simulink model "NeuromuscularModel"  (R2019b)
settings: Solver=ode15s  StartTime=0.0  StopTime=inf  MaxStep=.01  RelTol=1e-4  AbsTol=1e-6  EnableMultiTasking=on
values from neighbouring files (symbols this model uses):
  LceOffsetTA = 1-0.5*w    [ControlParams.m]
  legAngleTgt = 1.2    [ControlParams.m]    (also in assignGains.m = Gains(45))
  LongDelay = 0.020    (= 0.02)    [ControlParams.m]
  MidDelay = 0.010    (= 0.01)    [ControlParams.m]
  ShortDelay = 0.005    [ControlParams.m]
  simbiconGainD = 5*pi/180    (= 0.0872664625997)    [ControlParams.m]    (also in assignGains.m = Gains(42))
  simbiconGainV = 5*pi/180    (= 0.0872664625997)    [ControlParams.m]    (also in assignGains.m = Gains(43))
  simbiconLegAngle0 = 85*pi/180    (= 1.4835298642)    [ControlParams.m]    (also in assignGains.m = Gains(44))
undefined symbols (not defined in the file or in its folder): footCenterToCGDist, footInertia, footMass, g, legLengthClr, loptGAS, loptTA, lslackGAS, phimaxGASa, phimaxGASk, phirefGASa, phirefGASk, rGASa, rGASk, rhoGASa, rhoGASk, X, Y, Z
libraries: NeuroMuscularLibrary x81, nesl_utility x22, sm_lib x16, simulink x4, simulink_extras x2
(part 2 of 2)

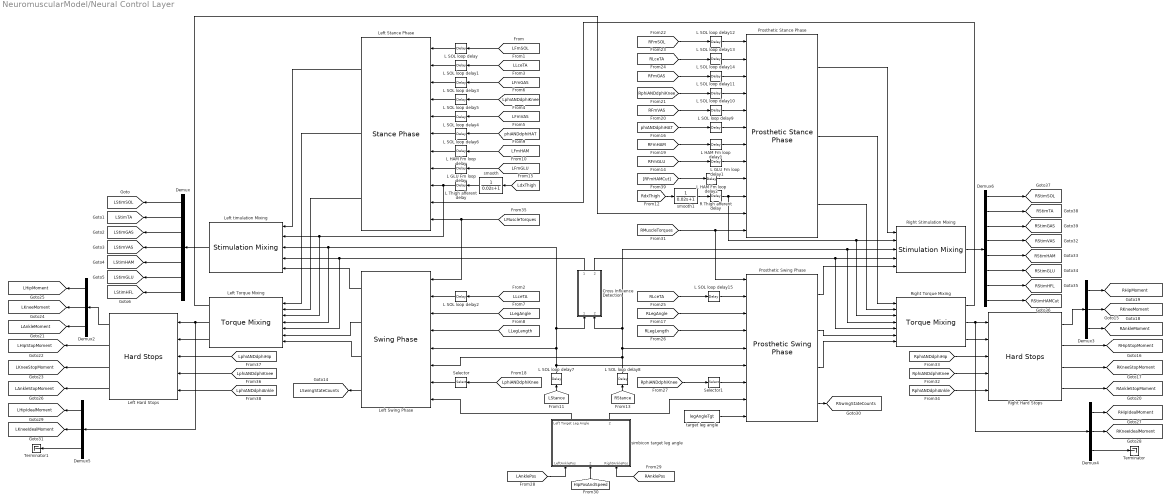
== system NeuromuscularModel/Neural Control Layer ==
  Cross Influence Detection : Subsystem
  Demux : Demux  Outputs=7
  Demux{2..5} (4 alike) : Demux  Outputs=3
  Demux6 : Demux  Outputs=8
  L GLU Fm loop delay : TransportDelay  DelayTime=ShortDelay
  L GLU Fm loop delay1 : TransportDelay  DelayTime=ShortDelay
  L HAM Fm loop delay : TransportDelay  DelayTime=ShortDelay
  L HAM Fm loop delay1 : TransportDelay  DelayTime=ShortDelay
  L HAM Fm loop delay2 : TransportDelay  DelayTime=ShortDelay  BufferSize=2048
  L SOL loop delay{,1..3,12..15} (8 alike) : TransportDelay  DelayTime=LongDelay
  L SOL loop delay{4..5,7..8,10..11} (6 alike) : TransportDelay  DelayTime=MidDelay
  L SOL loop delay6 : TransportDelay  DelayTime=ShortDelay
  L SOL loop delay9 : TransportDelay  DelayTime=ShortDelay
  L Thigh afferent delay : TransportDelay  DelayTime=ShortDelay
  Left Hard Stops : NeuroMuscularLibrary/Hard Stops  SystemSampleTime=-1  Latency=0  AutoFrameSizeCalculation=off
  Left Stance Phase : NeuroMuscularLibrary/Stance Phase  GainHAM=LGainHAM  GainGLU=LGainGLU  GainSOL=LGainSOL  GainSOLTA=LGainSOLTA  GainTA=LGainTA  GainGAS=LGainGAS  GainVAS=LGainVAS  GainKneeOverExt=LGainKneeOverExt  PosGainGG=LPosGainGG  SpeedGainGG=LSpeedGainGG  Kglu=LKglu
  Left Swing Phase : NeuroMuscularLibrary/Swing Phase  GainTA=LGainTA  hipPGain=LhipPGain  hipDGain=LhipDGain  legAngleFilter=LlegAngleFilter  kneeFlexGain=LkneeFlexGain  kneeHoldGain1=LkneeHoldGain1  kneeHoldGain2=LkneeHoldGain2  kneeStopGain=LkneeStopGain  kneeExtendGain=LkneeExtendGain  legLengthClr=LlegLengthClr
  Left Torque Mixing : NeuroMuscularLibrary/Torque Mixing  SystemSampleTime=-1  Latency=0  AutoFrameSizeCalculation=off
  Left timulation Mixing : NeuroMuscularLibrary/Stimulation Mixing  SystemSampleTime=-1  Latency=0  AutoFrameSizeCalculation=off
  Prosthetic Stance Phase : NeuroMuscularLibrary/Prosthetic Stance Phase  GainHAM=RGainHAM  GainHAMCut=RGainHAMCut  GainGLU=RGainGLU  GainSOL=RGainSOL  GainSOLTA=RGainSOLTA  GainTA=RGainTA  GainGAS=RGainGAS  GainVAS=RGainVAS  GainKneeOverExt=RGainKneeOverExt  PosGainGG=RPosGainGG  SpeedGainGG=RSpeedGainGG  Kglu=RKglu
  Prosthetic Swing Phase : NeuroMuscularLibrary/Prosthetic Swing Phase  GainTA=RGainTA  hipPGain=RhipPGain  hipDGain=RhipDGain  legAngleFilter=RlegAngleFilter  kneeFlexGain=RkneeFlexGain  kneeHoldGain1=RkneeHoldGain1  kneeHoldGain2=RkneeHoldGain2  kneeStopGain=RkneeStopGain  kneeExtendGain=RkneeExtendGain  legLengthClr=RlegLengthClr
  R Thigh afferent delay : TransportDelay  DelayTime=ShortDelay
  Right Hard Stops : NeuroMuscularLibrary/Hard Stops  SystemSampleTime=-1  Latency=0  AutoFrameSizeCalculation=off
  Right Stimulation Mixing : NeuroMuscularLibrary/Stimulation Mixing  SystemSampleTime=-1  Latency=0  AutoFrameSizeCalculation=off
  Right Torque Mixing : NeuroMuscularLibrary/Torque Mixing  SystemSampleTime=-1  Latency=0  AutoFrameSizeCalculation=off
  Selector : Selector  InputPortWidth=2  IndexOptions=Index vector (dialog)  Indices=2  OutputSizes=1
  Selector1 : Selector  InputPortWidth=2  IndexOptions=Index vector (dialog)  Indices=2  OutputSizes=1
  Terminator : Terminator
  Terminator1 : Terminator
  simbicon target leg angle : Subsystem
  smooth : TransferFcn  Denominator=[0.02 1]
  smooth1 : TransferFcn  Denominator=[0.02 1]
  target leg angle : Constant  Value=legAngleTgt
  tag scope: LAnkleMoment=global, LAnkleStopMoment=global, LHipIdealMoment=global, LHipMoment=global, LHipStopMoment=global, LKneeIdealMoment=global, LKneeMoment=global, LKneeStopMoment=global, LStimGAS=global, LStimGLU=global, LStimHAM=global, LStimHFL=global, LStimSOL=global, LStimTA=global, LStimVAS=global, LSwingStateCounts=global, RAnkleMoment=global, RAnkleStopMoment=global, RHipIdealMoment=global, RHipMoment=global, RHipStopMoment=global, RKneeIdealMoment=global, RKneeMoment=global, RKneeStopMoment=global, RStimGAS=global, RStimGLU=global, RStimHAM=global, RStimHAMCut=global, RStimHFL=global, RStimSOL=global, RStimTA=global, RStimVAS=global, RSwingStateCounts=global
  wires:
  target leg angle/1 -> Prosthetic Swing Phase/9
  L HAM Fm loop delay2/1 -> Prosthetic Stance Phase/9
  [RFmHAMCut] -> L HAM Fm loop delay2/1
  L GLU Fm loop delay1/1 -> Prosthetic Stance Phase/8
  L HAM Fm loop delay1/1 -> Prosthetic Stance Phase/7
  Demux6/8 -> [RStimHAMCut]
  Right Stimulation Mixing/1 -> Demux6/1
  Demux6/6 -> [RStimGLU]
  Demux6/3 -> [RStimGAS]
  Demux6/7 -> [RStimHFL]
  Demux6/5 -> [RStimHAM]
  Demux6/4 -> [RStimVAS]
  Demux6/2 -> [RStimTA]
  Demux6/1 -> [RStimSOL]
  Demux5/3 -> Terminator1/1
  Demux5/2 -> [LKneeIdealMoment]
  Demux5/1 -> [LHipIdealMoment]
  Left Swing Phase/3 -> Left Torque Mixing/7
  Left Swing Phase/2 -> Left Torque Mixing/6
  Left Stance Phase/3 -> Left Torque Mixing/2
  Left Torque Mixing/1 -> Prosthetic Stance Phase/11
  Left Torque Mixing/3 -> Left Hard Stops/2
  Left Torque Mixing/2 -> Left Hard Stops/1, Demux5/1
  [LphiANDdphiAnkle] -> Left Hard Stops/5
  Right Torque Mixing/1 -> Left Stance Phase/10
  Right Torque Mixing/3 -> Right Hard Stops/2
  Prosthetic Stance Phase/2 -> Right Torque Mixing/1
  Prosthetic Stance Phase/3 -> Right Torque Mixing/2
  Prosthetic Swing Phase/2 -> Right Torque Mixing/6
  Prosthetic Swing Phase/3 -> Right Torque Mixing/7
  Demux4/3 -> Terminator/1
  Demux4/2 -> [RKneeIdealMoment]
  Demux4/1 -> [RHipIdealMoment]
  [RMuscleTorques] -> Prosthetic Swing Phase/1, Prosthetic Stance Phase/12
  Right Hard Stops/1 -> Demux3/1
  Right Torque Mixing/2 -> Right Hard Stops/1, Demux4/1
  Demux2/2 -> [LKneeMoment]
  Left Stance Phase/2 -> Left Torque Mixing/1
  Left Hard Stops/4 -> [LAnkleStopMoment]
  Left Hard Stops/3 -> [LKneeStopMoment]
  Left Hard Stops/2 -> [LHipStopMoment]
  [LphiANDdphiHip] -> Left Hard Stops/3
  [LphiANDdphiKnee] -> Left Hard Stops/4
  Left Hard Stops/1 -> Demux2/1
  Demux2/3 -> [LAnkleMoment]
  Demux2/1 -> [LHipMoment]
  [LMuscleTorques] -> Left Stance Phase/11, Left Swing Phase/1
  Right Hard Stops/4 -> [RAnkleStopMoment]
  Right Hard Stops/3 -> [RKneeStopMoment]
  Right Hard Stops/2 -> [RHipStopMoment]
  [RphiANDdphiAnkle] -> Right Hard Stops/5
  [RphiANDdphiHip] -> Right Hard Stops/3
  [RphiANDdphiKnee] -> Right Hard Stops/4
  Demux3/3 -> [RAnkleMoment]
  Left Swing Phase/4 -> [LSwingStateCounts]
  Prosthetic Swing Phase/4 -> [RSwingStateCounts]
  simbicon target leg angle/1(Left Target Leg Angle) -> Left Swing Phase/8
  simbicon target leg angle/2(Right Target Leg Angle) -> Prosthetic Swing Phase/8
  [HipPosAndSpeed] -> simbicon target leg angle/2(HIPposAndSpeed)
  Left Swing Phase/1 -> Left timulation Mixing/5
  Selector/1 -> Left Swing Phase/7
  [LphiANDdphiKnee] -> Selector/1
  Prosthetic Swing Phase/1 -> Right Stimulation Mixing/5
  [RAnklePos] -> simbicon target leg angle/3(RightAnklePos)
  [LAnklePos] -> simbicon target leg angle/1(LeftAnklePos)
  Selector1/1 -> Prosthetic Swing Phase/7
  [RphiANDdphiKnee] -> Selector1/1
  [RLegLength] -> Prosthetic Swing Phase/4
  [RLegAngle] -> Prosthetic Swing Phase/3
  [LLegLength] -> Left Swing Phase/4
  [LLegAngle] -> Left Swing Phase/3
  Demux3/2 -> [RKneeMoment]
  Demux3/1 -> [RHipMoment]
  Cross Influence Detection/1(RightLeading) -> Left timulation Mixing/4, Left Torque Mixing/5
  Left Stance Phase/1 -> Left timulation Mixing/1
  Left timulation Mixing/1 -> Demux/1
  Cross Influence Detection/2(LeftLeading) -> Right Stimulation Mixing/4, Right Torque Mixing/5
  L SOL loop delay8/1 -> Cross Influence Detection/2(RStance), Right Stimulation Mixing/3, Right Torque Mixing/4, Prosthetic Swing Phase/5, Left Swing Phase/6
  Prosthetic Stance Phase/1 -> Right Stimulation Mixing/1
  L SOL loop delay2/1 -> Left Swing Phase/2
  L SOL loop delay15/1 -> Prosthetic Swing Phase/2
  R Thigh afferent delay/1 -> Right Stimulation Mixing/2, Right Torque Mixing/3, Prosthetic Stance Phase/10
  L GLU Fm loop delay/1 -> Left Stance Phase/8
  L HAM Fm loop delay/1 -> Left Stance Phase/7
  L Thigh afferent delay/1 -> Left Stance Phase/9, Left timulation Mixing/2, Left Torque Mixing/3
  [RLceTA] -> L SOL loop delay15/1
  L SOL loop delay14/1 -> Prosthetic Stance Phase/3
  [RFmGAS] -> L SOL loop delay14/1
  L SOL loop delay13/1 -> Prosthetic Stance Phase/2
  [RLceTA] -> L SOL loop delay13/1
  [RFmSOL] -> L SOL loop delay12/1
  L SOL loop delay12/1 -> Prosthetic Stance Phase/1
  L SOL loop delay11/1 -> Prosthetic Stance Phase/4
  L SOL loop delay10/1 -> Prosthetic Stance Phase/5
  [RphiANDdphiKnee] -> L SOL loop delay11/1
  [RFmVAS] -> L SOL loop delay10/1
  [RStance] -> L SOL loop delay8/1
  [LStance] -> L SOL loop delay7/1
  L SOL loop delay9/1 -> Prosthetic Stance Phase/6
  [phiANDdphiHAT] -> L SOL loop delay9/1
  [RFmGLU] -> L GLU Fm loop delay1/1
  [RFmHAM] -> L HAM Fm loop delay1/1
  L SOL loop delay7/1 -> Cross Influence Detection/1(LStance), Left timulation Mixing/3, Left Torque Mixing/4, Left Swing Phase/5, Prosthetic Swing Phase/6
  [LFmGLU] -> L GLU Fm loop delay/1
  [LFmHAM] -> L HAM Fm loop delay/1
  smooth1/1 -> R Thigh afferent delay/1
  [RdxThigh] -> smooth1/1
  smooth/1 -> L Thigh afferent delay/1
  [LdxThigh] -> smooth/1
  Demux/7 -> [LStimHFL]
  Demux/6 -> [LStimGLU]
  Demux/5 -> [LStimHAM]
  L SOL loop delay6/1 -> Left Stance Phase/6
  [phiANDdphiHAT] -> L SOL loop delay6/1
  Demux/4 -> [LStimVAS]
  [LphiANDdphiKnee] -> L SOL loop delay5/1
  L SOL loop delay5/1 -> Left Stance Phase/4
  [LFmVAS] -> L SOL loop delay4/1
  L SOL loop delay4/1 -> Left Stance Phase/5
  [LLceTA] -> L SOL loop delay2/1
  L SOL loop delay3/1 -> Left Stance Phase/3
  [LFmGAS] -> L SOL loop delay3/1
  Demux/3 -> [LStimGAS]
  Demux/2 -> [LStimTA]
  Demux/1 -> [LStimSOL]
  L SOL loop delay1/1 -> Left Stance Phase/2
  [LLceTA] -> L SOL loop delay1/1
  L SOL loop delay/1 -> Left Stance Phase/1
  [LFmSOL] -> L SOL loop delay/1

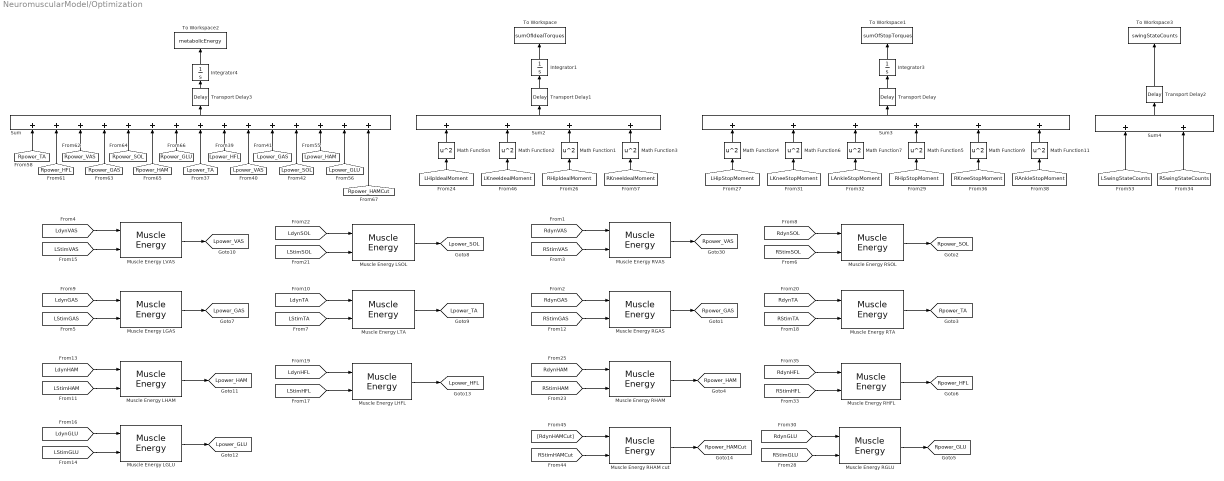
== system NeuromuscularModel/Optimization ==
  Integrator1 : Integrator
  Integrator3 : Integrator
  Integrator4 : Integrator
  Math Function{,1..7,9,11} (10 alike) : Math  Operator=square  SaturateOnIntegerOverflow=on
  Muscle Energy LGAS : NeuroMuscularLibrary/Muscle Energy  lopt=loptGAS  FT=FT_GAS  Fmax=FmaxGAS
  Muscle Energy LGLU : NeuroMuscularLibrary/Muscle Energy  lopt=loptGLU  FT=FT_GLU  Fmax=FmaxGLU
  Muscle Energy LHAM : NeuroMuscularLibrary/Muscle Energy  lopt=loptHAM  FT=FT_HAM  Fmax=FmaxHAM
  Muscle Energy LHFL : NeuroMuscularLibrary/Muscle Energy  lopt=loptHFL  FT=FT_HFL  Fmax=FmaxHFL
  Muscle Energy LSOL : NeuroMuscularLibrary/Muscle Energy  lopt=loptSOL  FT=FT_SOL  Fmax=FmaxSOL
  Muscle Energy LTA : NeuroMuscularLibrary/Muscle Energy  lopt=loptTA  FT=FT_TA  Fmax=FmaxTA
  Muscle Energy LVAS : NeuroMuscularLibrary/Muscle Energy  lopt=loptVAS  FT=FT_VAS  Fmax=FmaxVAS
  Muscle Energy RGAS : NeuroMuscularLibrary/Muscle Energy  lopt=loptGAS  FT=FT_GAS  Fmax=FmaxGAS
  Muscle Energy RGLU : NeuroMuscularLibrary/Muscle Energy  lopt=loptGLU  FT=FT_GLU  Fmax=FmaxGLU
  Muscle Energy RHAM : NeuroMuscularLibrary/Muscle Energy  lopt=loptHAM  FT=FT_HAM  Fmax=FmaxHAM
  Muscle Energy RHAM cut : NeuroMuscularLibrary/Muscle Energy  lopt=loptHAMCut  FT=FT_HAM  Fmax=FmaxHAMCut
  Muscle Energy RHFL : NeuroMuscularLibrary/Muscle Energy  lopt=loptHFL  FT=FT_HFL  Fmax=FmaxHFL
  Muscle Energy RSOL : NeuroMuscularLibrary/Muscle Energy  lopt=loptSOL  FT=FT_SOL  Fmax=FmaxSOL
  Muscle Energy RTA : NeuroMuscularLibrary/Muscle Energy  lopt=loptTA  FT=FT_TA  Fmax=FmaxTA
  Muscle Energy RVAS : NeuroMuscularLibrary/Muscle Energy  lopt=loptVAS  FT=FT_VAS  Fmax=FmaxVAS
  Sum : Sum  Inputs=+++++++++++++++
  Sum2 : Sum  Inputs=++++
  Sum3 : Sum  Inputs=++++++
  Sum4 : Sum
  To Workspace : ToWorkspace  VariableName=sumOfIdealTorques  SampleTime=-1
      settings: MaxDataPoints=1
  To Workspace1 : ToWorkspace  VariableName=sumOfStopTorques  SampleTime=-1
      settings: MaxDataPoints=1
  To Workspace2 : ToWorkspace  VariableName=metabolicEnergy  SampleTime=-1
      settings: MaxDataPoints=1
  To Workspace3 : ToWorkspace  VariableName=swingStateCounts  SampleTime=-1
      settings: MaxDataPoints=1
  Transport Delay{,1..3} (4 alike) : TransportDelay  DelayTime=3  BufferSize=24576
  tag scope: Lpower_GAS=global, Lpower_GLU=global, Lpower_HAM=global, Lpower_HFL=global, Lpower_SOL=global, Lpower_TA=global, Lpower_VAS=global, Rpower_GAS=global, Rpower_GLU=global, Rpower_HAM=global, Rpower_HAMCut=global, Rpower_HFL=global, Rpower_SOL=global, Rpower_TA=global, Rpower_VAS=global
  wires:
  [RdynSOL] -> Muscle Energy RSOL/1
  [RStimSOL] -> Muscle Energy RSOL/2
  [RStimVAS] -> Muscle Energy RVAS/2
  [RStimGAS] -> Muscle Energy RGAS/2
  Muscle Energy RVAS/1 -> [Rpower_VAS]
  Muscle Energy RGAS/1 -> [Rpower_GAS]
  Muscle Energy RSOL/1 -> [Rpower_SOL]
  Muscle Energy RTA/1 -> [Rpower_TA]
  [RdynTA] -> Muscle Energy RTA/1
  [RStimTA] -> Muscle Energy RTA/2
  [RdynHAM] -> Muscle Energy RHAM/1
  [RStimHAM] -> Muscle Energy RHAM/2
  [RdynGLU] -> Muscle Energy RGLU/1
  [RStimGLU] -> Muscle Energy RGLU/2
  [RdynHFL] -> Muscle Energy RHFL/1
  [RStimHFL] -> Muscle Energy RHFL/2
  Muscle Energy RHAM/1 -> [Rpower_HAM]
  Muscle Energy RGLU/1 -> [Rpower_GLU]
  Muscle Energy RHFL/1 -> [Rpower_HFL]
  [RdynGAS] -> Muscle Energy RGAS/1
  [RdynVAS] -> Muscle Energy RVAS/1
  [LdynSOL] -> Muscle Energy LSOL/1
  [LStimSOL] -> Muscle Energy LSOL/2
  [LStimVAS] -> Muscle Energy LVAS/2
  [LStimGAS] -> Muscle Energy LGAS/2
  Muscle Energy LVAS/1 -> [Lpower_VAS]
  Muscle Energy LGAS/1 -> [Lpower_GAS]
  Muscle Energy LSOL/1 -> [Lpower_SOL]
  Muscle Energy LTA/1 -> [Lpower_TA]
  [LdynTA] -> Muscle Energy LTA/1
  [LStimTA] -> Muscle Energy LTA/2
  [LdynHAM] -> Muscle Energy LHAM/1
  [LStimHAM] -> Muscle Energy LHAM/2
  [LdynGLU] -> Muscle Energy LGLU/1
  [LStimGLU] -> Muscle Energy LGLU/2
  [LdynHFL] -> Muscle Energy LHFL/1
  [LStimHFL] -> Muscle Energy LHFL/2
  Muscle Energy LHAM/1 -> [Lpower_HAM]
  Muscle Energy LGLU/1 -> [Lpower_GLU]
  Muscle Energy LHFL/1 -> [Lpower_HFL]
  [LdynGAS] -> Muscle Energy LGAS/1
  [LdynVAS] -> Muscle Energy LVAS/1
  [RdynHAMCut] -> Muscle Energy RHAM cut/1
  [RStimHAMCut] -> Muscle Energy RHAM cut/2
  Muscle Energy RHAM cut/1 -> [Rpower_HAMCut]
  Integrator1/1 -> To Workspace/1
  Math Function/1 -> Sum2/1
  [LHipIdealMoment] -> Math Function/1
  Math Function2/1 -> Sum2/2
  [LKneeIdealMoment] -> Math Function2/1
  [RHipIdealMoment] -> Math Function1/1
  Math Function1/1 -> Sum2/3
  [RKneeIdealMoment] -> Math Function3/1
  Math Function3/1 -> Sum2/4
  Integrator3/1 -> To Workspace1/1
  Math Function4/1 -> Sum3/1
  [LHipStopMoment] -> Math Function4/1
  Math Function6/1 -> Sum3/2
  [LKneeStopMoment] -> Math Function6/1
  [RHipStopMoment] -> Math Function5/1
  Math Function7/1 -> Sum3/3
  [LAnkleStopMoment] -> Math Function7/1
  Sum3/1 -> Transport Delay/1
  Transport Delay/1 -> Integrator3/1
  [RKneeStopMoment] -> Math Function9/1
  Math Function9/1 -> Sum3/5
  [RAnkleStopMoment] -> Math Function11/1
  Math Function11/1 -> Sum3/6
  Sum4/1 -> Transport Delay2/1
  Transport Delay2/1 -> To Workspace3/1
  [LSwingStateCounts] -> Sum4/1
  [RSwingStateCounts] -> Sum4/2
  [Rpower_TA] -> Sum/1
  [Rpower_GLU] -> Sum/7
  [Rpower_HAM] -> Sum/6
  [Rpower_SOL] -> Sum/5
  [Rpower_GAS] -> Sum/4
  [Rpower_VAS] -> Sum/3
  [Rpower_HFL] -> Sum/2
  [Lpower_TA] -> Sum/8
  [Lpower_GLU] -> Sum/14
  [Lpower_HAM] -> Sum/13
  [Lpower_SOL] -> Sum/12
  [Lpower_GAS] -> Sum/11
  [Lpower_VAS] -> Sum/10
  [Lpower_HFL] -> Sum/9
  Integrator4/1 -> To Workspace2/1
  Sum/1 -> Transport Delay3/1
  Transport Delay3/1 -> Integrator4/1
  [Rpower_HAMCut] -> Sum/15
  Sum2/1 -> Transport Delay1/1
  Transport Delay1/1 -> Integrator1/1
  Math Function5/1 -> Sum3/4

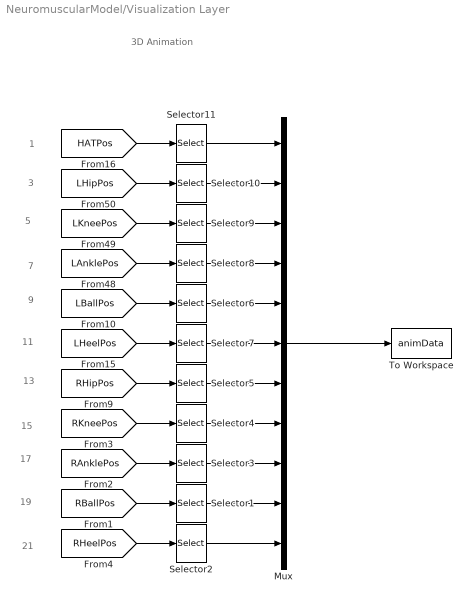
== system NeuromuscularModel/Visualization Layer ==
  note: 21
  note: 19
  note: 17
  note: 15
  note: 13
  note: 11
  note: 9
  note: 7
  note: 5
  note: 3
  note: 1
  note: 3D Animation
  Mux : Mux  Inputs=11
  Selector{1..11} (11 alike) : Selector  InputPortWidth=3  IndexOptions=Index vector (dialog)  Indices=[1 3]  OutputSizes=1
  To Workspace : ToWorkspace  VariableName=animData  SaveFormat=Structure With Time  SampleTime=1/30
  wires:
  [RAnklePos] -> Selector3/1
  [RKneePos] -> Selector4/1
  [RHipPos] -> Selector5/1
  [HATPos] -> Selector11/1
  [LHeelPos] -> Selector7/1
  [LBallPos] -> Selector6/1
  [LAnklePos] -> Selector8/1
  [LKneePos] -> Selector9/1
  [LHipPos] -> Selector10/1
  Selector11/1 -> Mux/1
  Selector3/1 -> Mux/9
  Selector4/1 -> Mux/8
  Selector5/1 -> Mux/7
  Selector7/1 -> Mux/6
  Selector6/1 -> Mux/5
  Selector8/1 -> Mux/4
  Selector9/1 -> Mux/3
  Selector10/1 -> Mux/2
  Mux/1 -> To Workspace/1
  [RHeelPos] -> Selector2/1
  [RBallPos] -> Selector1/1
  Selector2/1 -> Mux/11
  Selector1/1 -> Mux/10

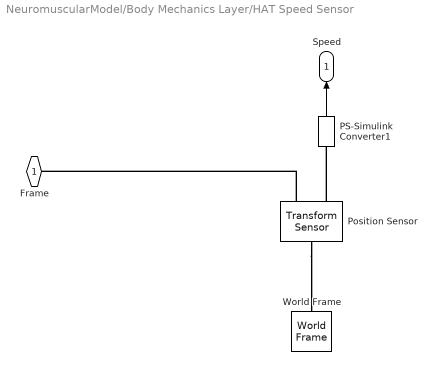
== system NeuromuscularModel/Body Mechanics Layer/HAT Speed Sensor ==
  PS-Simulink Converter1 : nesl_utility/PS-Simulink Converter  PhysicalDomain=network_engine_domain  SubClassName=ps_output  LeftPortType=input  RightPortType=output  PseudoPeriodic=off  Frequencies=[]  Unit=m/s  AffineConversion=off
  Position Sensor : sm_lib/Frames and Transforms/Transform Sensor  MeasurementFrame=World  SenseAngle=off  SenseAxis=off  SenseAngle1=off  SenseAngle2=off  SenseAngle3=off  SenseQ=off  SenseR=off  SenseOmegaX=off  SenseOmegaY=off  SenseOmegaZ=off  SenseOmega1=off  SenseOmega2=off  SenseOmega3=off  SenseQDot=off  SenseRDot=off  SenseAlphaX=off  SenseAlphaY=off  SenseAlphaZ=off  SenseAlpha1=off  SenseAlpha2=off  SenseAlpha3=off  SenseQDDot=off  SenseRDDot=off  SenseX=off  SenseY=off  SenseZ=off  SenseRad=off  SenseAzim=off  SenseDist=off  SenseInc=off  SenseXDot=on  SenseYDot=off  SenseZDot=off  SenseRadDot=off  SenseAzimDot=off  SenseDistDot=off  SenseIncDot=off  SenseXDDot=off  SenseYDDot=off  SenseZDDot=off  SenseRadDDot=off  SenseAzimDDot=off  SenseDistDDot=off  SenseIncDDot=off
  World Frame : sm_lib/Frames and Transforms/World Frame
  Frame : PMIOPort  Side=Left
  Speed : Outport
  wires:
  PS-Simulink Converter1/1 -> Speed/1
  connections:
  Position Sensor/LConn1 -- World Frame/RConn1
  Position Sensor/RConn1 -- Frame/RConn1
  Position Sensor/RConn2 -- PS-Simulink Converter1/LConn1

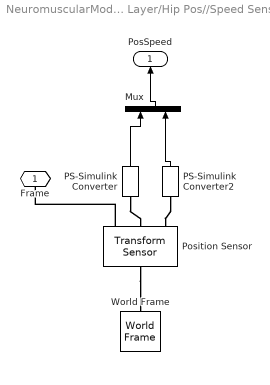
== system NeuromuscularModel/Body Mechanics Layer/Hip Pos//Speed Sensor ==
  Mux : Mux  Inputs=2
  PS-Simulink Converter : nesl_utility/PS-Simulink Converter  PhysicalDomain=network_engine_domain  SubClassName=ps_output  LeftPortType=input  RightPortType=output  PseudoPeriodic=off  Frequencies=[]  Unit=m  AffineConversion=off
  PS-Simulink Converter2 : nesl_utility/PS-Simulink Converter  PhysicalDomain=network_engine_domain  SubClassName=ps_output  LeftPortType=input  RightPortType=output  PseudoPeriodic=off  Frequencies=[]  Unit=m/s  AffineConversion=off
  Position Sensor : sm_lib/Frames and Transforms/Transform Sensor  MeasurementFrame=World  SenseAngle=off  SenseAxis=off  SenseAngle1=off  SenseAngle2=off  SenseAngle3=off  SenseQ=off  SenseR=off  SenseOmegaX=off  SenseOmegaY=off  SenseOmegaZ=off  SenseOmega1=off  SenseOmega2=off  SenseOmega3=off  SenseQDot=off  SenseRDot=off  SenseAlphaX=off  SenseAlphaY=off  SenseAlphaZ=off  SenseAlpha1=off  SenseAlpha2=off  SenseAlpha3=off  SenseQDDot=off  SenseRDDot=off  SenseX=on  SenseY=off  SenseZ=off  SenseRad=off  SenseAzim=off  SenseDist=off  SenseInc=off  SenseXDot=on  SenseYDot=off  SenseZDot=off  SenseRadDot=off  SenseAzimDot=off  SenseDistDot=off  SenseIncDot=off  SenseXDDot=off  SenseYDDot=off  SenseZDDot=off  SenseRadDDot=off  SenseAzimDDot=off  SenseDistDDot=off  SenseIncDDot=off
  World Frame : sm_lib/Frames and Transforms/World Frame
  Frame : PMIOPort  Side=Left
  PosSpeed : Outport
  wires:
  Mux/1 -> PosSpeed/1
  PS-Simulink Converter/1 -> Mux/1
  PS-Simulink Converter2/1 -> Mux/2
  connections:
  Position Sensor/LConn1 -- World Frame/RConn1
  Position Sensor/RConn1 -- Frame/RConn1
  PS-Simulink Converter/LConn1 -- Position Sensor/RConn2
  PS-Simulink Converter2/LConn1 -- Position Sensor/RConn3

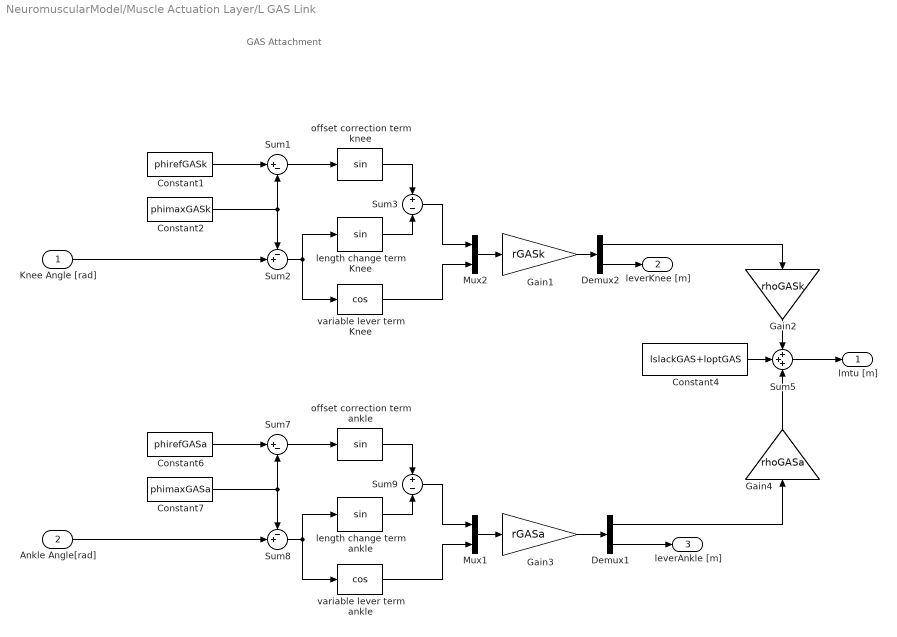
== system NeuromuscularModel/Muscle Actuation Layer/L GAS Link ==
  note: GAS Attachment
  Knee Angle [rad] : Inport
  Ankle Angle[rad] : Inport  Port=2
  Constant1 : Constant  Value=phirefGASk
  Constant2 : Constant  Value=phimaxGASk
  Constant4 : Constant  Value=lslackGAS+loptGAS
  Constant6 : Constant  Value=phirefGASa
  Constant7 : Constant  Value=phimaxGASa
  Demux1 : Demux  Outputs=2
  Demux2 : Demux  Outputs=2
  Gain1 : Gain  Gain=rGASk
  Gain2 : Gain  Gain=rhoGASk
  Gain3 : Gain  Gain=rGASa
  Gain4 : Gain  Gain=rhoGASa
  Mux1 : Mux  Inputs=2
  Mux2 : Mux  Inputs=2
  Sum1 : Sum  Inputs=|+-
  Sum2 : Sum  Inputs=-+|
  Sum3 : Sum  Inputs=+-
  Sum5 : Sum  Inputs=+++
  Sum7 : Sum  Inputs=|+-
  Sum8 : Sum  Inputs=-+|
  Sum9 : Sum  Inputs=+-
  length change term Knee : Trigonometry
  length change term ankle : Trigonometry
  offset correction term ankle : Trigonometry
  offset correction term knee : Trigonometry
  variable lever term Knee : Trigonometry  Operator=cos
  variable lever term ankle : Trigonometry  Operator=cos
  lmtu [m] : Outport
  leverKnee [m] : Outport  Port=2
  leverAnkle [m] : Outport  Port=3
  wires:
  Ankle Angle[rad]/1 -> Sum8/2
  Sum5/1 -> lmtu [m]/1
  variable lever term ankle/1 -> Mux1/2
  Demux1/2 -> leverAnkle [m]/1
  Sum8/1 -> variable lever term ankle/1, length change term ankle/1
  Constant7/1 -> Sum8/1, Sum7/2
  Sum7/1 -> offset correction term ankle/1
  Constant6/1 -> Sum7/1
  length change term ankle/1 -> Sum9/2
  offset correction term ankle/1 -> Sum9/1
  Sum9/1 -> Mux1/1
  Constant4/1 -> Sum5/2
  Mux1/1 -> Gain3/1
  Gain3/1 -> Demux1/1
  Demux1/1 -> Gain4/1
  Gain4/1 -> Sum5/3
  Knee Angle [rad]/1 -> Sum2/2
  variable lever term Knee/1 -> Mux2/2
  Sum2/1 -> variable lever term Knee/1, length change term Knee/1
  Constant2/1 -> Sum2/1, Sum1/2
  Sum1/1 -> offset correction term knee/1
  Constant1/1 -> Sum1/1
  length change term Knee/1 -> Sum3/2
  offset correction term knee/1 -> Sum3/1
  Sum3/1 -> Mux2/1
  Mux2/1 -> Gain1/1
  Gain1/1 -> Demux2/1
  Demux2/2 -> leverKnee [m]/1
  Demux2/1 -> Gain2/1
  Gain2/1 -> Sum5/1

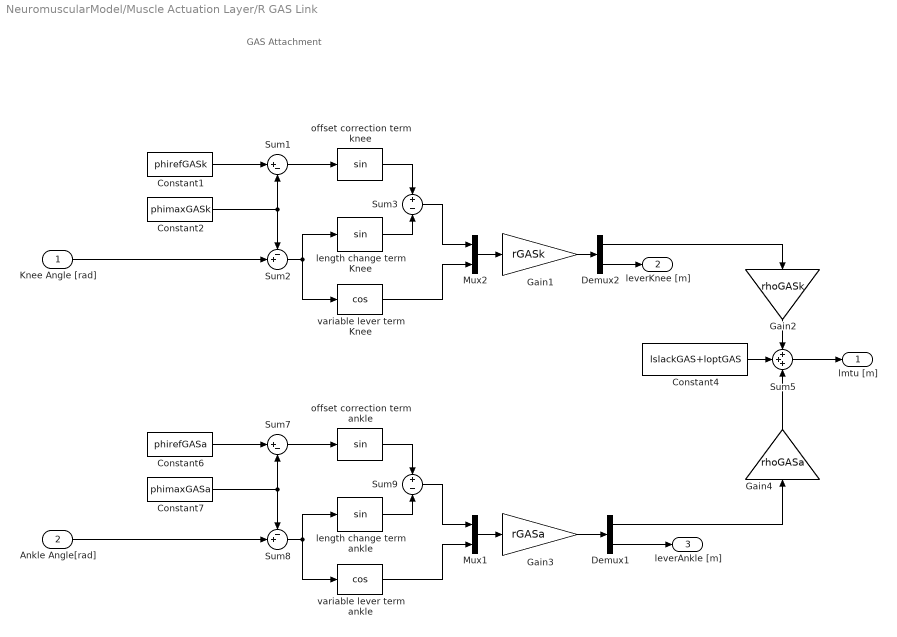
== system NeuromuscularModel/Muscle Actuation Layer/R GAS Link ==
  note: GAS Attachment
  Knee Angle [rad] : Inport
  Ankle Angle[rad] : Inport  Port=2
  Constant1 : Constant  Value=phirefGASk
  Constant2 : Constant  Value=phimaxGASk
  Constant4 : Constant  Value=lslackGAS+loptGAS
  Constant6 : Constant  Value=phirefGASa
  Constant7 : Constant  Value=phimaxGASa
  Demux1 : Demux  Outputs=2
  Demux2 : Demux  Outputs=2
  Gain1 : Gain  Gain=rGASk
  Gain2 : Gain  Gain=rhoGASk
  Gain3 : Gain  Gain=rGASa
  Gain4 : Gain  Gain=rhoGASa
  Mux1 : Mux  Inputs=2
  Mux2 : Mux  Inputs=2
  Sum1 : Sum  Inputs=|+-
  Sum2 : Sum  Inputs=-+|
  Sum3 : Sum  Inputs=+-
  Sum5 : Sum  Inputs=+++
  Sum7 : Sum  Inputs=|+-
  Sum8 : Sum  Inputs=-+|
  Sum9 : Sum  Inputs=+-
  length change term Knee : Trigonometry
  length change term ankle : Trigonometry
  offset correction term ankle : Trigonometry
  offset correction term knee : Trigonometry
  variable lever term Knee : Trigonometry  Operator=cos
  variable lever term ankle : Trigonometry  Operator=cos
  lmtu [m] : Outport
  leverKnee [m] : Outport  Port=2
  leverAnkle [m] : Outport  Port=3
  wires:
  Ankle Angle[rad]/1 -> Sum8/2
  Sum5/1 -> lmtu [m]/1
  variable lever term ankle/1 -> Mux1/2
  Demux1/2 -> leverAnkle [m]/1
  Sum8/1 -> variable lever term ankle/1, length change term ankle/1
  Constant7/1 -> Sum8/1, Sum7/2
  Sum7/1 -> offset correction term ankle/1
  Constant6/1 -> Sum7/1
  length change term ankle/1 -> Sum9/2
  offset correction term ankle/1 -> Sum9/1
  Sum9/1 -> Mux1/1
  Constant4/1 -> Sum5/2
  Mux1/1 -> Gain3/1
  Gain3/1 -> Demux1/1
  Demux1/1 -> Gain4/1
  Gain4/1 -> Sum5/3
  Knee Angle [rad]/1 -> Sum2/2
  variable lever term Knee/1 -> Mux2/2
  Sum2/1 -> variable lever term Knee/1, length change term Knee/1
  Constant2/1 -> Sum2/1, Sum1/2
  Sum1/1 -> offset correction term knee/1
  Constant1/1 -> Sum1/1
  length change term Knee/1 -> Sum3/2
  offset correction term knee/1 -> Sum3/1
  Sum3/1 -> Mux2/1
  Mux2/1 -> Gain1/1
  Gain1/1 -> Demux2/1
  Demux2/2 -> leverKnee [m]/1
  Demux2/1 -> Gain2/1
  Gain2/1 -> Sum5/1

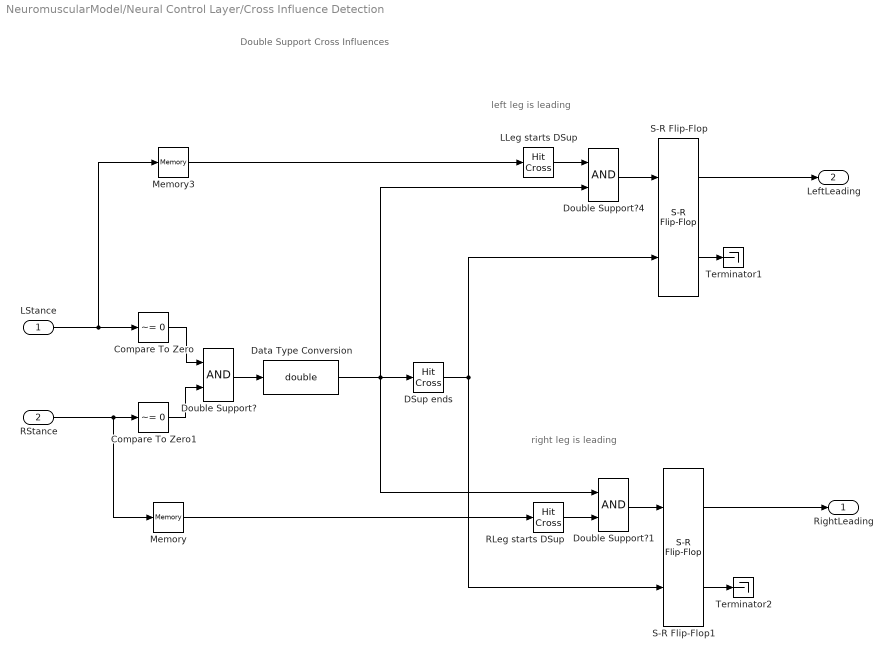
== system NeuromuscularModel/Neural Control Layer/Cross Influence Detection ==
  note: Double Support Cross Influences
  note: left leg is leading
  note: right leg is leading
  LStance : Inport
  RStance : Inport  Port=2
  Compare To Zero : simulink/Logic and Bit Operations/Compare To Zero  relop=~=  OutDataTypeStr=boolean
  Compare To Zero1 : simulink/Logic and Bit Operations/Compare To Zero  relop=~=  OutDataTypeStr=boolean
  DSup ends : HitCross  HitCrossingOffset=0.5  HitCrossingDirection=falling  ZeroCross=off
  Data Type Conversion : DataTypeConversion  OutDataTypeStr=double
  Double Support? : Logic  AllPortsSameDT=off
  Double Support?1 : Logic  AllPortsSameDT=off
  Double Support?4 : Logic  AllPortsSameDT=off
  LLeg starts DSup : HitCross  HitCrossingOffset=0.5  HitCrossingDirection=rising  ZeroCross=off
  Memory : Memory
  Memory3 : Memory
  RLeg starts DSup : HitCross  HitCrossingOffset=0.5  HitCrossingDirection=rising  ZeroCross=off
  S-R Flip-Flop : simulink_extras/Flip Flops/S-R Flip-Flop  initial_condition=0
  S-R Flip-Flop1 : simulink_extras/Flip Flops/S-R Flip-Flop  initial_condition=0
  Terminator1 : Terminator
  Terminator2 : Terminator
  RightLeading : Outport
  LeftLeading : Outport  Port=2
  wires:
  Data Type Conversion/1 -> DSup ends/1, Double Support?4/2, Double Support?1/1
  Double Support?/1 -> Data Type Conversion/1
  Compare To Zero1/1 -> Double Support?/2
  Compare To Zero/1 -> Double Support?/1
  DSup ends/1 -> S-R Flip-Flop1/2, S-R Flip-Flop/2
  Double Support?4/1 -> S-R Flip-Flop/1
  LLeg starts DSup/1 -> Double Support?4/1
  Memory3/1 -> LLeg starts DSup/1
  Double Support?1/1 -> S-R Flip-Flop1/1
  RLeg starts DSup/1 -> Double Support?1/2
  Memory/1 -> RLeg starts DSup/1
  S-R Flip-Flop1/1 -> RightLeading/1
  RStance/1 -> Memory/1, Compare To Zero1/1
  LStance/1 -> Compare To Zero/1, Memory3/1
  S-R Flip-Flop1/2 -> Terminator2/1
  S-R Flip-Flop/1 -> LeftLeading/1
  S-R Flip-Flop/2 -> Terminator1/1

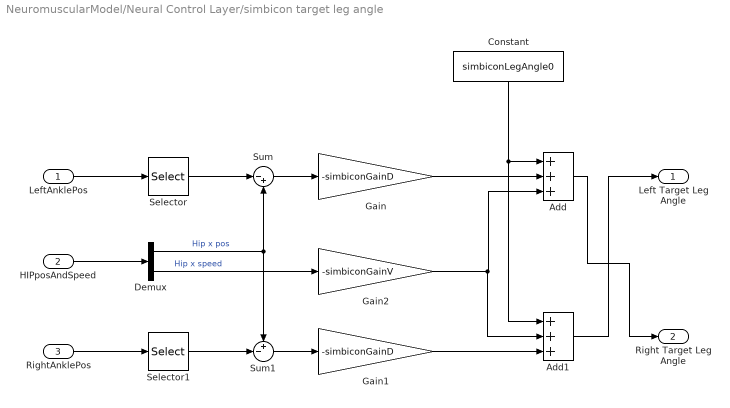
== system NeuromuscularModel/Neural Control Layer/simbicon target leg angle ==
  LeftAnklePos : Inport
  HIPposAndSpeed : Inport  Port=2
  RightAnklePos : Inport  Port=3
  Add : Sum  Inputs=+++
  Add1 : Sum  Inputs=+++
  Constant : Constant  Value=simbiconLegAngle0
  Demux : Demux  Outputs=2
  Gain : Gain  Gain=-simbiconGainD
  Gain1 : Gain  Gain=-simbiconGainD
  Gain2 : Gain  Gain=-simbiconGainV
  Selector : Selector  InputPortWidth=3  IndexOptions=Index vector (dialog)  Indices=[1]  OutputSizes=1
  Selector1 : Selector  InputPortWidth=3  IndexOptions=Index vector (dialog)  Indices=[1]  OutputSizes=1
  Sum : Sum  Inputs=|-+
  Sum1 : Sum  Inputs=+-|
  Left Target Leg Angle : Outport
  Right Target Leg Angle : Outport  Port=2
  wires:
  Demux/2 -> Gain2/1  "Hip x speed"
  Selector1/1 -> Sum1/2
  RightAnklePos/1 -> Selector1/1
  Selector/1 -> Sum/1
  LeftAnklePos/1 -> Selector/1
  Add/1 -> Right Target Leg Angle/1
  Add1/1 -> Left Target Leg Angle/1
  Constant/1 -> Add1/1, Add/1
  Gain1/1 -> Add1/3
  Gain2/1 -> Add/3, Add1/2
  Gain/1 -> Add/2
  Sum1/1 -> Gain1/1
  Sum/1 -> Gain/1
  Demux/1 -> Sum1/1, Sum/2  "Hip x pos"
  HIPposAndSpeed/1 -> Demux/1
